simulink model "simulink_progetto"  (R2024a)
settings: Solver=VariableStepAuto  StartTime=0.0  StopTime=10.0  RelTol=1e-3
undefined symbols (not defined in the file): denominatore_cs, denominatore_eulero_avanti, denominatore_eulero_indietro, denominatore_ps, numeratore_cs, numeratore_eulero_avanti, numeratore_eulero_indietro, numeratore_ps, Ts
settings Model: Creator=franc  LastModifiedBy=franc

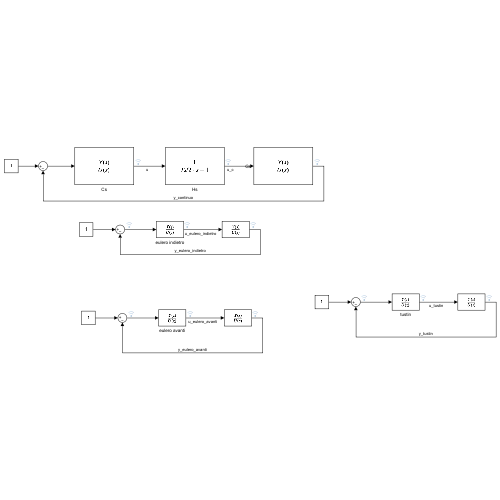
[thumbnail: Simulink's stored preview of the top-level diagram]
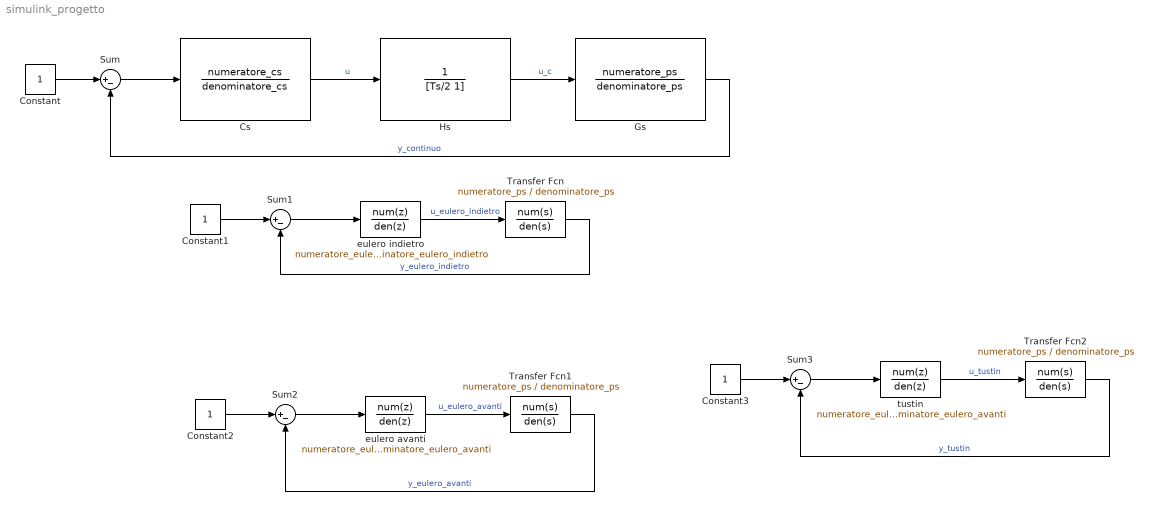
== system simulink_progetto ==
  Constant{,1..3} (4 alike) : Constant
  Cs : TransferFcn  Numerator=numeratore_cs  Denominator=denominatore_cs
  Gs : TransferFcn  Numerator=numeratore_ps  Denominator=denominatore_ps
  Hs : TransferFcn  Numerator=1  Denominator=[Ts/2 1]
  Sum{,1..3} (4 alike) : Sum  Inputs=|+-
  Transfer Fcn : TransferFcn  Numerator=numeratore_ps  Denominator=denominatore_ps
  Transfer Fcn1 : TransferFcn  Numerator=numeratore_ps  Denominator=denominatore_ps
  Transfer Fcn2 : TransferFcn  Numerator=numeratore_ps  Denominator=denominatore_ps
  eulero avanti : DiscreteTransferFcn  Numerator=numeratore_eulero_avanti  Denominator=denominatore_eulero_avanti
  eulero indietro : DiscreteTransferFcn  Numerator=numeratore_eulero_indietro  Denominator=denominatore_eulero_indietro
  tustin : DiscreteTransferFcn  Numerator=numeratore_eulero_avanti  Denominator=denominatore_eulero_avanti
  wires:
  Hs/1 -> Gs/1  "u_c"
  Cs/1 -> Hs/1  "u"
  Gs/1 -> Sum/2  "y_continuo"
  Constant/1 -> Sum/1
  Sum/1 -> Cs/1
  Constant1/1 -> Sum1/1
  Sum1/1 -> eulero indietro/1
  eulero indietro/1 -> Transfer Fcn/1  "u_eulero_indietro"
  Transfer Fcn/1 -> Sum1/2  "y_eulero_indietro"
  Constant2/1 -> Sum2/1
  eulero avanti/1 -> Transfer Fcn1/1  "u_eulero_avanti"
  Transfer Fcn1/1 -> Sum2/2  "y_eulero_avanti"
  Sum2/1 -> eulero avanti/1
  Sum3/1 -> tustin/1
  tustin/1 -> Transfer Fcn2/1  "u_tustin"
  Transfer Fcn2/1 -> Sum3/2  "y_tustin"
  Constant3/1 -> Sum3/1
